simulink model "sampleModel1540"  (R2023a)
settings: Solver=VariableStepAuto  StartTime=0.0  StopTime=10.0  RelTol=1e-3
libraries: hdlsllib x5, simulink x4
settings Model: Creator=user1  LastModifiedBy=user1

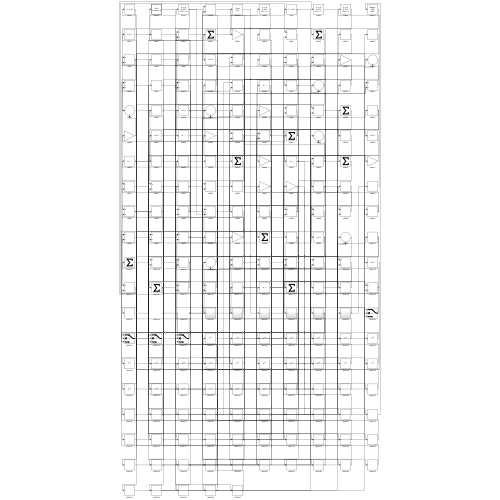
[thumbnail: Simulink's stored preview of the top-level diagram]
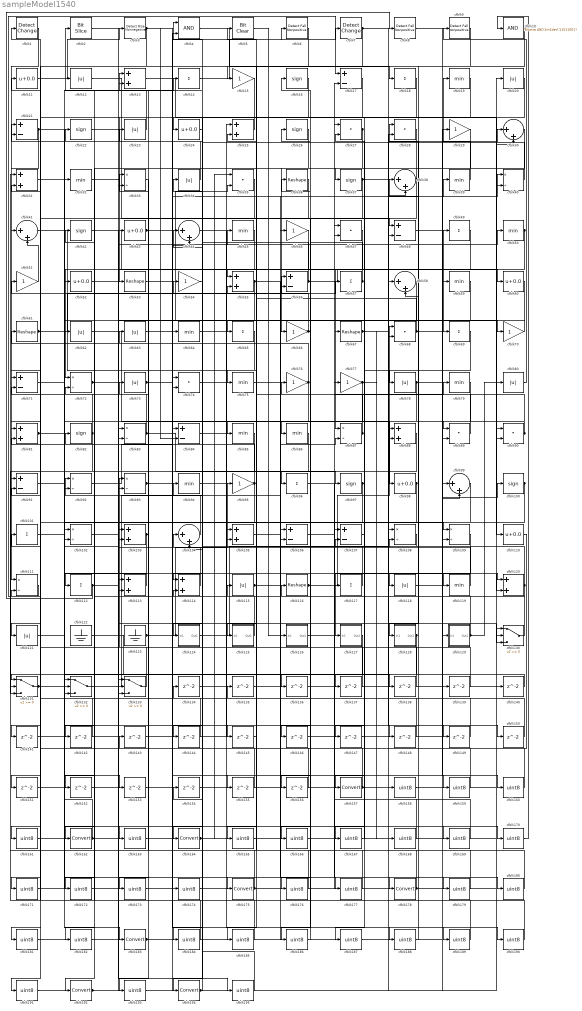
== system sampleModel1540 ==
  cfblk1 : simulink/Logic and Bit Operations/Detect Change  vinit=0  OutDataTypeStr=boolean
      settings: LibrarySourceBlock=|
      | hdlsllib/Logic and Bit
      | Operations/Detect
      | Change
  cfblk10 : simulink/Logic and Bit Operations/Bitwise Operator  logicop=AND  UseBitMask=on  BitMask=bin2dec('11011001')  BitMaskRealWorld=Stored Integer
      settings: LibrarySourceBlock=|
      | hdlsllib/Logic and Bit
      | Operations/Bitwise
      | Operator
  cfblk{16,22,26,37,42,82,97,100} (8 alike) : Signum
  cfblk{14,18,49,57,65,69,96,101,112,117} (10 alike) : Sum  Inputs=+
  cfblk{33,40,72,83,87,92..93,102,108..109,111} (11 alike) : Product  Inputs=*/  RndMeth=Zero  SaturateOnIntegerOverflow=on
  cfblk{13,25,31,55,81,88,103,105,113..114,120} (11 alike) : Sum
  cfblk{30,38,41,44,58,99,104} (7 alike) : Sum  Inputs=|++
  cfblk{17,21,48,56,71,84,91,106..107} (9 alike) : Sum  Inputs=+-
  cfblk{11,24,43,52,60,98,110} (7 alike) : Bias  Bias=0.0  SaturateOnIntegerOverflow=off
  cfblk{12,20,23,34,62..63,73,78,80,115,118,121} (12 alike) : Abs  SaturateOnIntegerOverflow=off
  cfblk{36,53,61,67,116} (5 alike) : Reshape
  cfblk{19,32,39,45,50,59,64,75,79,85..86,94,119} (13 alike) : MinMax
  cfblk122 : Ground
  cfblk123 : Ground
  cfblk124 : Subsystem
      settings: LibrarySourceBlock=|
      | hdlsllib/Ports &
      | Subsystems/Subsystem
  cfblk125 : Subsystem
      settings: LibrarySourceBlock=|
      | hdlsllib/Ports &
      | Subsystems/Subsystem
  cfblk126 : Subsystem
      settings: LibrarySourceBlock=|
      | hdlsllib/Ports &
      | Subsystems/Subsystem
  cfblk127 : Subsystem
      settings: LibrarySourceBlock=|
      | hdlsllib/Ports &
      | Subsystems/Subsystem
  cfblk128 : Subsystem
      settings: LibrarySourceBlock=|
      | hdlsllib/Ports &
      | Subsystems/Subsystem
  cfblk129 : Subsystem
      settings: LibrarySourceBlock=|
      | hdlsllib/Ports &
      | Subsystems/Subsystem
  cfblk{130..133} (4 alike) : Switch  SaturateOnIntegerOverflow=off  InputSameDT=off
  cfblk{134..156} (23 alike) : Delay  SampleTime=1
  cfblk{15,29,46,51,54,66,70,76..77,95} (10 alike) : Gain
  cfblk{157,162,164,175,178,183,192,194} (8 alike) : DataTypeConversion  SaturateOnIntegerOverflow=off  RndMeth=Floor
  cfblk{158..161,163,165..174,176..177,179..182,184..191,193,195} (31 alike) : DataTypeConversion  OutDataTypeStr=uint8  SaturateOnIntegerOverflow=off  RndMeth=Floor
  cfblk2 : hdlsllib/Logic and Bit Operations/Bit Slice  lidx=7  ridx=0
  cfblk{27..28,35,47,68,74,89..90} (8 alike) : DotProduct  OutDataTypeStr=Inherit: Inherit via internal rule
  cfblk3 : hdlsllib/Logic and Bit Operations/Detect Rise Nonnegative  vinit=0  OutDataTypeStr=boolean
  cfblk4 : Logic  AllPortsSameDT=off  OutDataTypeStr=boolean
  cfblk5 : simulink/Logic and Bit Operations/Bit Clear  iBit=0
      settings: LibrarySourceBlock=|
      | hdlsllib/Logic and Bit
      | Operations/Bit Clear
  cfblk6 : hdlsllib/Logic and Bit Operations/Detect Fall Nonpositive  vinit=0  OutDataTypeStr=boolean
  cfblk7 : simulink/Logic and Bit Operations/Detect Change  vinit=0  OutDataTypeStr=boolean
      settings: LibrarySourceBlock=|
      | hdlsllib/Logic and Bit
      | Operations/Detect
      | Change
  cfblk8 : hdlsllib/Logic and Bit Operations/Detect Fall Nonpositive  vinit=0  OutDataTypeStr=boolean
  cfblk9 : hdlsllib/Logic and Bit Operations/Detect Fall Nonpositive  vinit=0  OutDataTypeStr=boolean
  wires:
  cfblk1/1 -> cfblk111/1
  cfblk5/1 -> cfblk126/1(In1)
  cfblk15/1 -> cfblk53/1
  cfblk68/1 -> cfblk25/2, cfblk160/1
  cfblk83/1 -> cfblk97/1, cfblk12/1
  cfblk114/1 -> cfblk104/1
  cfblk21/1 -> cfblk41/1, cfblk145/1
  cfblk94/1 -> cfblk178/1
  cfblk116/1 -> cfblk68/1, cfblk120/1, cfblk79/1
  cfblk92/1 -> cfblk64/1
  cfblk48/1 -> cfblk69/1
  cfblk129/1(Out1) -> cfblk80/1, cfblk42/1
  cfblk42/1 -> cfblk87/1
  cfblk34/1 -> cfblk22/1
  cfblk56/1 -> cfblk60/1, cfblk13/2
  cfblk80/1 -> cfblk9/1
  cfblk97/1 -> cfblk146/1, cfblk187/1
  cfblk111/1 -> cfblk17/1
  cfblk78/1 -> cfblk130/2, cfblk136/1
  cfblk112/1 -> cfblk8/1, cfblk195/1
  cfblk63/1 -> cfblk45/1
  cfblk26/1 -> cfblk66/1
  cfblk39/1 -> cfblk19/1
  cfblk31/1 -> cfblk183/1
  cfblk14/1 -> cfblk7/1
  cfblk27/1 -> cfblk65/1, cfblk33/2
  cfblk86/1 -> cfblk121/1
  cfblk4/1 -> cfblk18/1
  cfblk11/1 -> cfblk3/1
  cfblk12/1 -> cfblk48/1
  cfblk61/1 -> cfblk56/1, cfblk120/2
  cfblk133/1 -> cfblk93/1
  cfblk57/1 -> cfblk55/1, cfblk26/1
  cfblk64/1 -> cfblk96/1
  cfblk16/1 -> cfblk131/1
  cfblk115/1 -> cfblk87/2, cfblk40/1
  cfblk132/1 -> cfblk56/2
  cfblk96/1 -> cfblk119/1
  cfblk73/1 -> cfblk6/1, cfblk13/1
  cfblk62/1 -> cfblk98/1
  cfblk30/1 -> cfblk75/1
  cfblk72/1 -> cfblk130/3, cfblk152/1
  cfblk123/1 -> cfblk95/1, cfblk73/1, cfblk190/1
  cfblk99/1 -> cfblk164/1
  cfblk119/1 -> cfblk103/1
  cfblk117/1 -> cfblk76/1
  cfblk126/1(Out1) -> cfblk77/1
  cfblk38/1 -> cfblk37/1, cfblk166/1
  cfblk103/1 -> cfblk23/1, cfblk113/2
  cfblk67/1 -> cfblk109/2, cfblk158/1
  cfblk25/1 -> cfblk24/1
  cfblk45/1 -> cfblk72/1
  cfblk29/1 -> cfblk192/1
  cfblk131/1 -> cfblk103/2, cfblk137/1
  cfblk59/1 -> cfblk128/1(In1)
  cfblk46/1 -> cfblk162/1
  cfblk9/1 -> cfblk85/1
  cfblk77/1 -> cfblk92/2, cfblk168/1
  cfblk52/1 -> cfblk70/1
  cfblk18/1 -> cfblk81/1
  cfblk109/1 -> cfblk127/1(In1)
  cfblk102/1 -> cfblk50/1
  cfblk87/1 -> cfblk36/1, cfblk86/1
  cfblk10/1 -> cfblk78/1
  cfblk124/1(Out1) -> cfblk108/2
  cfblk17/1 -> cfblk124/1(In1)
  cfblk128/1(Out1) -> cfblk141/1, cfblk181/1
  cfblk89/1 -> cfblk5/1
  cfblk118/1 -> cfblk100/1
  cfblk105/1 -> cfblk57/1
  cfblk130/1 -> cfblk16/1
  cfblk91/1 -> cfblk175/1
  cfblk65/1 -> cfblk83/2
  cfblk125/1(Out1) -> cfblk82/1
  cfblk95/1 -> cfblk33/1, cfblk51/1, cfblk191/1
  cfblk82/1 -> cfblk11/1, cfblk131/3
  cfblk40/1 -> cfblk4/1
  cfblk120/1 -> cfblk21/1, cfblk114/2
  cfblk41/1 -> cfblk113/1
  cfblk93/1 -> cfblk40/2, cfblk148/1
  cfblk54/1 -> cfblk194/1
  cfblk113/1 -> cfblk112/1
  cfblk70/1 -> cfblk62/1
  cfblk104/1 -> cfblk92/1
  cfblk20/1 -> cfblk67/1
  cfblk75/1 -> cfblk118/1
  cfblk51/1 -> cfblk41/2
  cfblk50/1 -> cfblk117/1, cfblk156/1
  cfblk7/1 -> cfblk15/1, cfblk150/1
  cfblk55/1 -> cfblk132/3, cfblk179/1
  cfblk22/1 -> cfblk59/1
  cfblk3/1 -> cfblk84/2, cfblk71/1, cfblk155/1
  cfblk43/1 -> cfblk90/2, cfblk35/2
  cfblk23/1 -> cfblk2/1
  cfblk121/1 -> cfblk52/1
  cfblk6/1 -> cfblk93/2
  cfblk13/1 -> cfblk110/1
  cfblk66/1 -> cfblk21/2, cfblk176/1
  cfblk98/1 -> cfblk104/2, cfblk132/2
  cfblk49/1 -> cfblk157/1
  cfblk108/1 -> cfblk105/2
  cfblk100/1 -> cfblk125/1(In1), cfblk173/1
  cfblk76/1 -> cfblk61/1, cfblk114/1
  cfblk79/1 -> cfblk88/1
  cfblk37/1 -> cfblk30/1, cfblk102/2
  cfblk81/1 -> cfblk14/1, cfblk109/1, cfblk177/1
  cfblk90/1 -> cfblk89/1, cfblk28/1
  cfblk84/1 -> cfblk39/1
  cfblk134/1 -> cfblk17/2
  cfblk135/1 -> cfblk90/1
  cfblk136/1 -> cfblk27/1
  cfblk137/1 -> cfblk1/1
  cfblk2/1 -> cfblk138/1
  cfblk138/1 -> cfblk105/1
  cfblk8/1 -> cfblk139/1
  cfblk139/1 -> cfblk108/1
  cfblk140/1 -> cfblk131/2
  cfblk141/1 -> cfblk25/1
  cfblk60/1 -> cfblk142/1
  cfblk142/1 -> cfblk132/1
  cfblk110/1 -> cfblk143/1
  cfblk35/1 -> cfblk144/1
  cfblk144/1 -> cfblk83/1
  cfblk145/1 -> cfblk55/2
  cfblk146/1 -> cfblk89/2
  cfblk69/1 -> cfblk147/1
  cfblk147/1 -> cfblk48/2
  cfblk148/1 -> cfblk133/1
  cfblk53/1 -> cfblk149/1
  cfblk149/1 -> cfblk81/2
  cfblk150/1 -> cfblk133/2
  cfblk127/1(Out1) -> cfblk151/1
  cfblk151/1 -> cfblk4/2
  cfblk152/1 -> cfblk38/2
  cfblk101/1 -> cfblk153/1
  cfblk154/1 -> cfblk30/2
  cfblk155/1 -> cfblk111/2
  cfblk156/1 -> cfblk71/2
  cfblk157/1 -> cfblk101/1, cfblk84/1
  cfblk158/1 -> cfblk49/1
  cfblk74/1 -> cfblk159/1
  cfblk159/1 -> cfblk134/1
  cfblk160/1 -> cfblk74/1
  cfblk88/1 -> cfblk161/1
  cfblk161/1 -> cfblk74/2
  cfblk162/1 -> cfblk88/2, cfblk102/1
  cfblk71/1 -> cfblk163/1
  cfblk163/1 -> cfblk46/1
  cfblk164/1 -> cfblk130/1, cfblk35/1
  cfblk28/1 -> cfblk165/1
  cfblk165/1 -> cfblk99/1
  cfblk166/1 -> cfblk99/2
  cfblk107/1 -> cfblk167/1
  cfblk167/1 -> cfblk27/2
  cfblk168/1 -> cfblk107/1
  cfblk153/1 -> cfblk169/1
  cfblk169/1 -> cfblk107/2
  cfblk32/1 -> cfblk170/1
  cfblk170/1 -> cfblk10/1
  cfblk36/1 -> cfblk171/1
  cfblk171/1 -> cfblk32/1
  cfblk47/1 -> cfblk172/1
  cfblk172/1 -> cfblk43/1
  cfblk173/1 -> cfblk47/1
  cfblk122/1 -> cfblk174/1
  cfblk174/1 -> cfblk47/2
  cfblk175/1 -> cfblk154/1, cfblk20/1, cfblk63/1
  cfblk176/1 -> cfblk91/1
  cfblk177/1 -> cfblk91/2
  cfblk178/1 -> cfblk115/1, cfblk38/1
  cfblk179/1 -> cfblk94/1
  cfblk106/1 -> cfblk180/1
  cfblk180/1 -> cfblk135/1
  cfblk181/1 -> cfblk106/1
  cfblk85/1 -> cfblk182/1
  cfblk182/1 -> cfblk106/2
  cfblk183/1 -> cfblk28/2, cfblk129/1(In1)
  cfblk24/1 -> cfblk184/1
  cfblk184/1 -> cfblk31/1
  cfblk19/1 -> cfblk185/1
  cfblk185/1 -> cfblk31/2
  cfblk58/1 -> cfblk186/1
  cfblk186/1 -> cfblk116/1
  cfblk187/1 -> cfblk58/1
  cfblk143/1 -> cfblk188/1
  cfblk188/1 -> cfblk58/2
  cfblk44/1 -> cfblk189/1
  cfblk189/1 -> cfblk72/2
  cfblk190/1 -> cfblk44/1
  cfblk191/1 -> cfblk44/2
  cfblk192/1 -> cfblk133/3, cfblk68/2
  cfblk33/1 -> cfblk193/1
  cfblk193/1 -> cfblk29/1
  cfblk194/1 -> cfblk140/1, cfblk34/1
  cfblk195/1 -> cfblk54/1

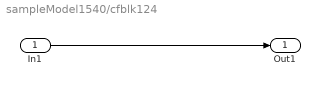
== system sampleModel1540/cfblk124 ==
  In1 : Inport
  Out1 : Outport
  wires:
  In1/1 -> Out1/1

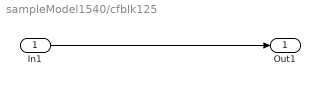
== system sampleModel1540/cfblk125 ==
  In1 : Inport
  Out1 : Outport
  wires:
  In1/1 -> Out1/1

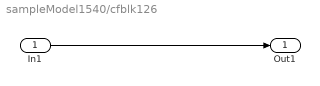
== system sampleModel1540/cfblk126 ==
  In1 : Inport
  Out1 : Outport
  wires:
  In1/1 -> Out1/1

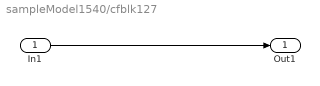
== system sampleModel1540/cfblk127 ==
  In1 : Inport
  Out1 : Outport
  wires:
  In1/1 -> Out1/1

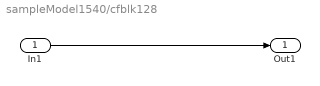
== system sampleModel1540/cfblk128 ==
  In1 : Inport
  Out1 : Outport
  wires:
  In1/1 -> Out1/1

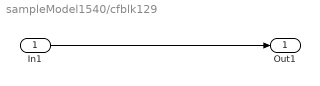
== system sampleModel1540/cfblk129 ==
  In1 : Inport
  Out1 : Outport
  wires:
  In1/1 -> Out1/1
